simulink model "Purchase"  (R2015a)
settings: Solver=FixedStepDiscrete  StartTime=0.0  StopTime=1000  FixedStep=0.1  RelTol=1e-3
libraries: simulink x1
settings Model: Creator=higashit  LastModifiedBy=aohashi
settings SolverCC: AlgebraicLoopSolver=LineSearch
settings DataIOCC: SaveOutput=off  SaveTime=off
settings OptimizationCC: ExpressionDepthLimit=2147483647  EfficientFloat2IntCast=on
settings DebuggingCC: SolverPrmCheckMsg=warning  UniqueDataStoreMsg=error  StateNameClashWarn=warning  StrictBusMsg=ErrorOnBusTreatedAsVector
settings ConfigComp: Description=Design Verifier Custom Configuration Component  DVMaxTestCaseSteps=500  DVTestSuiteOptimization=CombinedObjectives (Nonlinear Extended)

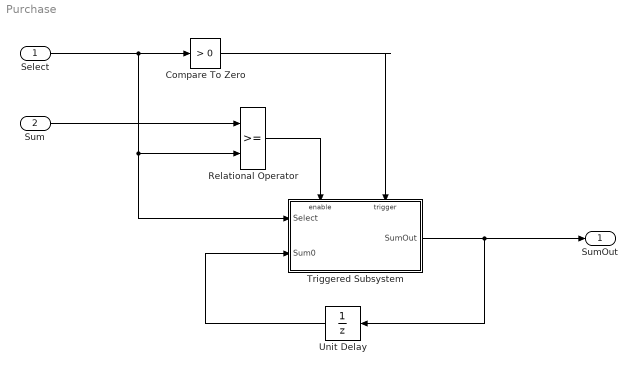
== system Purchase ==
  Select : Inport  OutDataTypeStr=uint16  PortDimensions=1
  Sum : Inport  Port=2  OutDataTypeStr=uint16  PortDimensions=1
  Compare To Zero : simulink/Logic and Bit Operations/Compare To Zero  relop=>  OutDataTypeStr=boolean
  Relational Operator : RelationalOperator  OutDataTypeStr=boolean
  Triggered Subsystem : Subsystem  TreatAsAtomicUnit=on
  Unit Delay : UnitDelay  SampleTime=-1
  SumOut : Outport  OutDataTypeStr=uint16  PortDimensions=1
  wires:
  Sum/1 -> Relational Operator/1
  Triggered Subsystem/1(SumOut) -> SumOut/1, Unit Delay/1
  Relational Operator/1 -> Triggered Subsystem/Enable
  Compare To Zero/1 -> Triggered Subsystem/Trigger
  Select/1 -> Triggered Subsystem/1(Select), Relational Operator/2, Compare To Zero/1
  Unit Delay/1 -> Triggered Subsystem/2(Sum0)

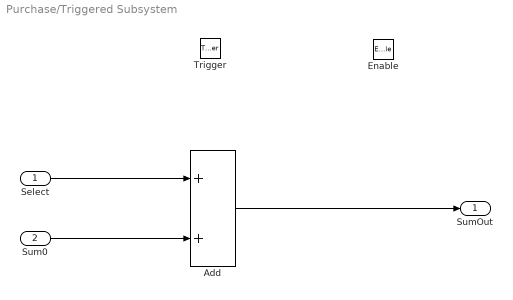
== system Purchase/Triggered Subsystem ==
  Select : Inport
  Sum0 : Inport  Port=2
  Enable : EnablePort
  Trigger : TriggerPort
  Add : Sum  OutDataTypeStr=uint16
  SumOut : Outport  InitialOutput=0
  wires:
  Sum0/1 -> Add/2
  Add/1 -> SumOut/1
  Select/1 -> Add/1
